simulink model "dsp_blr_hikaku_nakamura_futagi"  (R2018a)
settings: Solver=VariableStepAuto  StartTime=0.0  StopTime=100e-6  RelTol=1e-3
values from neighbouring files (symbols this model uses):
  BASELINE = 0    [dsp_blr.mat]
libraries: xbsIndex_r4 x934, xrbsSSR_Library x35, simulink x3, dspsigattribs x2, hdlsllib x2
(part 2 of 6)

== system dsp_blr_hikaku_nakamura_futagi/+cut ==
  In1 : Inport
  AddSub7 : xbsIndex_r4/AddSub  mode=Subtraction  use_carryin=off  use_carryout=off  en=off  latency=0  precision=User Defined  arith_type="Signed  (2's comp)"  n_bits=17  bin_pt=4  quantization=Truncate  overflow=Wrap  use_behavioral_HDL=off  hw_selection=Fabric  pipelined=off  dbl_ovrd=off  block_type=addsub
  Delay2 : xbsIndex_r4/Delay  rst=off  infoeditControl=Selection of Reset will increase slice count due to use of real FFs and instead of SRLs  en=off  latency=1  reg_retiming=off  dbl_ovrd=off  block_type=delay
  Delay3 : xbsIndex_r4/Delay  rst=off  infoeditControl=Selection of Reset will increase slice count due to use of real FFs and instead of SRLs  en=off  latency=3  reg_retiming=off  dbl_ovrd=off  block_type=delay
  P*e[n] : xbsIndex_r4/Mult  precision=Full  arith_type="Signed  (2's comp)"  n_bits=16  bin_pt=14  quantization=Truncate  overflow=Wrap  en=off  latency=3  use_behavioral_HDL=off  opt=Speed  use_embedded=on  optimum_pipeline=off  pipeline=on  dbl_ovrd=off  use_rpm=on  placement_style=Triangular  block_type=mult
  Shift7 : xbsIndex_r4/Shift  shift_dir=Right  shift_bits=1  en=off  latency=1  precision=Full  arith_type="Signed  (2's comp)"  n_bits=16  bin_pt=14  quantization=Truncate  overflow=Wrap  dbl_ovrd=off  block_type=shift
  Threshold : xbsIndex_r4/Threshold  en=off  latency=1  dbl_ovrd=off  block_type=sgn
      settings: infoedit="Presents -1 as output if input is negative; otherwise presents 1.  Output is a two bit signed number."
  Out1 : Outport
  wires:
  Shift7/1 -> Out1/1
  Delay2/1 -> P*e[n]/1, Delay3/1
  In1/1 -> Threshold/1, Delay2/1
  Threshold/1 -> P*e[n]/2
  Delay3/1 -> AddSub7/1
  AddSub7/1 -> Shift7/1
  P*e[n]/1 -> AddSub7/2

== system dsp_blr_hikaku_nakamura_futagi/8sample_average 1 ==
  valid_in : Inport
  data_in : Inport  Port=2
  Vector_sum : Subsystem
  scaling : Subsystem
  ave_valid_out : Outport
  ave_data_out : Outport  Port=2
  wires:
  valid_in/1 -> scaling/1(valid_in)
  Vector_sum/1(sum_data_out) -> scaling/2(data_in)
  scaling/2(data_out) -> ave_data_out/1
  data_in/1 -> Vector_sum/1(tdata_in)
  scaling/1(valid_out) -> ave_valid_out/1

== system dsp_blr_hikaku_nakamura_futagi/8sample_average 3 ==
  valid_in : Inport
  data_in : Inport  Port=2
  Vector_sum : Subsystem
  scaling : Subsystem
  ave_valid_out : Outport
  ave_data_out : Outport  Port=2
  wires:
  valid_in/1 -> scaling/1(valid_in)
  Vector_sum/1(sum_data_out) -> scaling/2(data_in)
  scaling/2(data_out) -> ave_data_out/1
  data_in/1 -> Vector_sum/1(tdata_in)
  scaling/1(valid_out) -> ave_valid_out/1

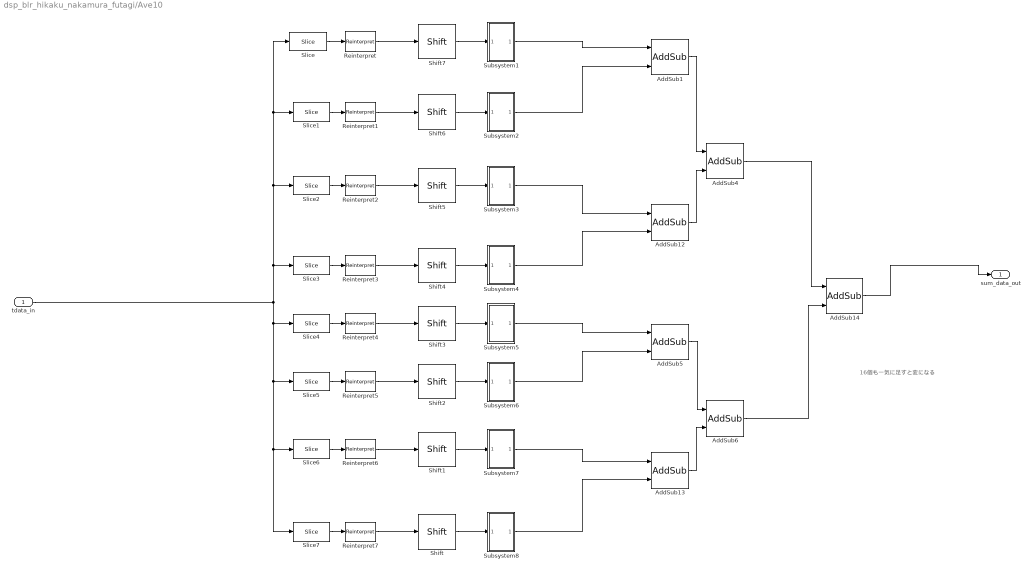
== system dsp_blr_hikaku_nakamura_futagi/Ave10 ==
  note: 16個も一気に足すと変になる
  tdata_in : Inport
  AddSub{1,12..14} (4 alike) : xbsIndex_r4/AddSub  mode=Addition  use_carryin=off  use_carryout=off  en=off  latency=0  precision=User Defined  arith_type="Signed  (2's comp)"  n_bits=17  bin_pt=4  quantization=Truncate  overflow=Wrap  use_behavioral_HDL=off  hw_selection=Fabric  pipelined=off  dbl_ovrd=off  block_type=addsub
  AddSub4 : xbsIndex_r4/AddSub  mode=Addition  use_carryin=off  use_carryout=off  en=off  latency=0  precision=Full  arith_type="Signed  (2's comp)"  n_bits=18  bin_pt=4  quantization=Truncate  overflow=Wrap  use_behavioral_HDL=off  hw_selection=Fabric  pipelined=off  dbl_ovrd=off  block_type=addsub
  AddSub5 : xbsIndex_r4/AddSub  mode=Addition  use_carryin=off  use_carryout=off  en=off  latency=0  precision=Full  arith_type="Signed  (2's comp)"  n_bits=18  bin_pt=4  quantization=Truncate  overflow=Wrap  use_behavioral_HDL=off  hw_selection=Fabric  pipelined=off  dbl_ovrd=off  block_type=addsub
  AddSub6 : xbsIndex_r4/AddSub  mode=Addition  use_carryin=off  use_carryout=off  en=off  latency=0  precision=User Defined  arith_type="Signed  (2's comp)"  n_bits=19  bin_pt=4  quantization=Truncate  overflow=Wrap  use_behavioral_HDL=off  hw_selection=Fabric  pipelined=off  dbl_ovrd=off  block_type=addsub
  Reinterpret{,1..7} (8 alike) : xbsIndex_r4/Reinterpret  force_arith_type=on  arith_type="Signed  (2's comp)"  force_bin_pt=on  bin_pt=4  block_type=reinterpret
  Shift{,1..7} (8 alike) : xbsIndex_r4/Shift  shift_dir=Right  shift_bits=6  en=off  latency=1  precision=Full  arith_type="Signed  (2's comp)"  n_bits=16  bin_pt=14  quantization=Truncate  overflow=Wrap  dbl_ovrd=off  block_type=shift
  Slice : xbsIndex_r4/Slice  nbits=16  boolean_output=off  mode=Two Bit Locations  bit1=15  base1=LSB of Input  bit0=0  base0=LSB of Input  dbl_ovrd=off  block_type=slice
  Slice1 : xbsIndex_r4/Slice  nbits=16  boolean_output=off  mode=Two Bit Locations  bit1=31  base1=LSB of Input  bit0=16  base0=LSB of Input  dbl_ovrd=off  block_type=slice
  Slice2 : xbsIndex_r4/Slice  nbits=16  boolean_output=off  mode=Two Bit Locations  bit1=47  base1=LSB of Input  bit0=32  base0=LSB of Input  dbl_ovrd=off  block_type=slice
  Slice3 : xbsIndex_r4/Slice  nbits=16  boolean_output=off  mode=Two Bit Locations  bit1=63  base1=LSB of Input  bit0=48  base0=LSB of Input  dbl_ovrd=off  block_type=slice
  Slice4 : xbsIndex_r4/Slice  nbits=16  boolean_output=off  mode=Two Bit Locations  bit1=79  base1=LSB of Input  bit0=64  base0=LSB of Input  dbl_ovrd=off  block_type=slice
  Slice5 : xbsIndex_r4/Slice  nbits=16  boolean_output=off  mode=Two Bit Locations  bit1=95  base1=LSB of Input  bit0=80  base0=LSB of Input  dbl_ovrd=off  block_type=slice
  Slice6 : xbsIndex_r4/Slice  nbits=16  boolean_output=off  mode=Two Bit Locations  bit1=111  base1=LSB of Input  bit0=96  base0=LSB of Input  dbl_ovrd=off  block_type=slice
  Slice7 : xbsIndex_r4/Slice  nbits=16  boolean_output=off  mode=Two Bit Locations  bit1=127  base1=LSB of Input  bit0=112  base0=LSB of Input  dbl_ovrd=off  block_type=slice
  Subsystem1 : Subsystem
  Subsystem2 : Subsystem
  Subsystem3 : Subsystem
  Subsystem4 : Subsystem
  Subsystem5 : Subsystem
  Subsystem6 : Subsystem
  Subsystem7 : Subsystem
  Subsystem8 : Subsystem
  sum_data_out : Outport  OutDataTypeStr=fixdt(1,19,4)
  wires:
  AddSub14/1 -> sum_data_out/1
  Reinterpret5/1 -> Shift2/1
  Reinterpret4/1 -> Shift3/1
  Reinterpret7/1 -> Shift/1
  Reinterpret3/1 -> Shift4/1
  Reinterpret2/1 -> Shift5/1
  Reinterpret1/1 -> Shift6/1
  Reinterpret/1 -> Shift7/1
  Slice7/1 -> Reinterpret7/1
  Slice6/1 -> Reinterpret6/1
  Slice5/1 -> Reinterpret5/1
  Slice4/1 -> Reinterpret4/1
  Slice3/1 -> Reinterpret3/1
  Slice2/1 -> Reinterpret2/1
  Slice1/1 -> Reinterpret1/1
  Slice/1 -> Reinterpret/1
  Subsystem5/1(Out1) -> AddSub5/1
  Subsystem6/1(Out1) -> AddSub5/2
  tdata_in/1 -> Slice3/1, Slice1/1, Slice/1, Slice2/1, Slice4/1, Slice5/1, Slice6/1, Slice7/1
  Reinterpret6/1 -> Shift1/1
  Subsystem3/1(Out1) -> AddSub12/1
  Subsystem4/1(Out1) -> AddSub12/2
  Subsystem7/1(Out1) -> AddSub13/1
  Subsystem8/1(Out1) -> AddSub13/2
  AddSub13/1 -> AddSub6/2
  AddSub5/1 -> AddSub6/1
  AddSub1/1 -> AddSub4/1
  AddSub12/1 -> AddSub4/2
  AddSub4/1 -> AddSub14/1
  AddSub6/1 -> AddSub14/2
  Shift/1 -> Subsystem8/1(In1)
  Shift1/1 -> Subsystem7/1(In1)
  Shift2/1 -> Subsystem6/1(In1)
  Shift3/1 -> Subsystem5/1(In1)
  Shift4/1 -> Subsystem4/1(In1)
  Shift5/1 -> Subsystem3/1(In1)
  Shift6/1 -> Subsystem2/1(In1)
  Shift7/1 -> Subsystem1/1(In1)
  Subsystem1/1(Out1) -> AddSub1/1
  Subsystem2/1(Out1) -> AddSub1/2

== system dsp_blr_hikaku_nakamura_futagi/Ave11 ==
  note: 16個も一気に足すと変になる
  tdata_in : Inport
  AddSub14 : xbsIndex_r4/AddSub  mode=Addition  use_carryin=off  use_carryout=off  en=off  latency=0  precision=User Defined  arith_type="Signed  (2's comp)"  n_bits=17  bin_pt=4  quantization=Truncate  overflow=Wrap  use_behavioral_HDL=off  hw_selection=Fabric  pipelined=off  dbl_ovrd=off  block_type=addsub
  AddSub4 : xbsIndex_r4/AddSub  mode=Addition  use_carryin=off  use_carryout=off  en=off  latency=0  precision=Full  arith_type="Signed  (2's comp)"  n_bits=18  bin_pt=4  quantization=Truncate  overflow=Wrap  use_behavioral_HDL=off  hw_selection=Fabric  pipelined=off  dbl_ovrd=off  block_type=addsub
  AddSub6 : xbsIndex_r4/AddSub  mode=Addition  use_carryin=off  use_carryout=off  en=off  latency=0  precision=User Defined  arith_type="Signed  (2's comp)"  n_bits=19  bin_pt=4  quantization=Truncate  overflow=Wrap  use_behavioral_HDL=off  hw_selection=Fabric  pipelined=off  dbl_ovrd=off  block_type=addsub
  Reinterpret{,2,4,6} (4 alike) : xbsIndex_r4/Reinterpret  force_arith_type=on  arith_type="Signed  (2's comp)"  force_bin_pt=on  bin_pt=4  block_type=reinterpret
  Shift{2,4,6..7} (4 alike) : xbsIndex_r4/Shift  shift_dir=Right  shift_bits=6  en=off  latency=1  precision=Full  arith_type="Signed  (2's comp)"  n_bits=16  bin_pt=14  quantization=Truncate  overflow=Wrap  dbl_ovrd=off  block_type=shift
  Slice : xbsIndex_r4/Slice  nbits=16  boolean_output=off  mode=Two Bit Locations  bit1=15  base1=LSB of Input  bit0=0  base0=LSB of Input  dbl_ovrd=off  block_type=slice
  Slice2 : xbsIndex_r4/Slice  nbits=16  boolean_output=off  mode=Two Bit Locations  bit1=47  base1=LSB of Input  bit0=32  base0=LSB of Input  dbl_ovrd=off  block_type=slice
  Slice4 : xbsIndex_r4/Slice  nbits=16  boolean_output=off  mode=Two Bit Locations  bit1=79  base1=LSB of Input  bit0=64  base0=LSB of Input  dbl_ovrd=off  block_type=slice
  Slice6 : xbsIndex_r4/Slice  nbits=16  boolean_output=off  mode=Two Bit Locations  bit1=111  base1=LSB of Input  bit0=96  base0=LSB of Input  dbl_ovrd=off  block_type=slice
  Subsystem1 : Subsystem
  Subsystem3 : Subsystem
  Subsystem5 : Subsystem
  Subsystem7 : Subsystem
  sum_data_out : Outport  OutDataTypeStr=fixdt(1,19,4)
  wires:
  AddSub14/1 -> sum_data_out/1
  Reinterpret4/1 -> Shift4/1
  Reinterpret2/1 -> Shift2/1
  Reinterpret/1 -> Shift7/1
  Slice6/1 -> Reinterpret6/1
  Slice4/1 -> Reinterpret4/1
  Slice2/1 -> Reinterpret2/1
  Slice/1 -> Reinterpret/1
  tdata_in/1 -> Slice/1, Slice2/1, Slice4/1, Slice6/1
  Reinterpret6/1 -> Shift6/1
  Subsystem7/1(Out1) -> AddSub6/2
  Subsystem5/1(Out1) -> AddSub6/1
  Subsystem1/1(Out1) -> AddSub4/1
  Subsystem3/1(Out1) -> AddSub4/2
  AddSub4/1 -> AddSub14/1
  AddSub6/1 -> AddSub14/2
  Shift6/1 -> Subsystem7/1(In1)
  Shift4/1 -> Subsystem5/1(In1)
  Shift2/1 -> Subsystem3/1(In1)
  Shift7/1 -> Subsystem1/1(In1)

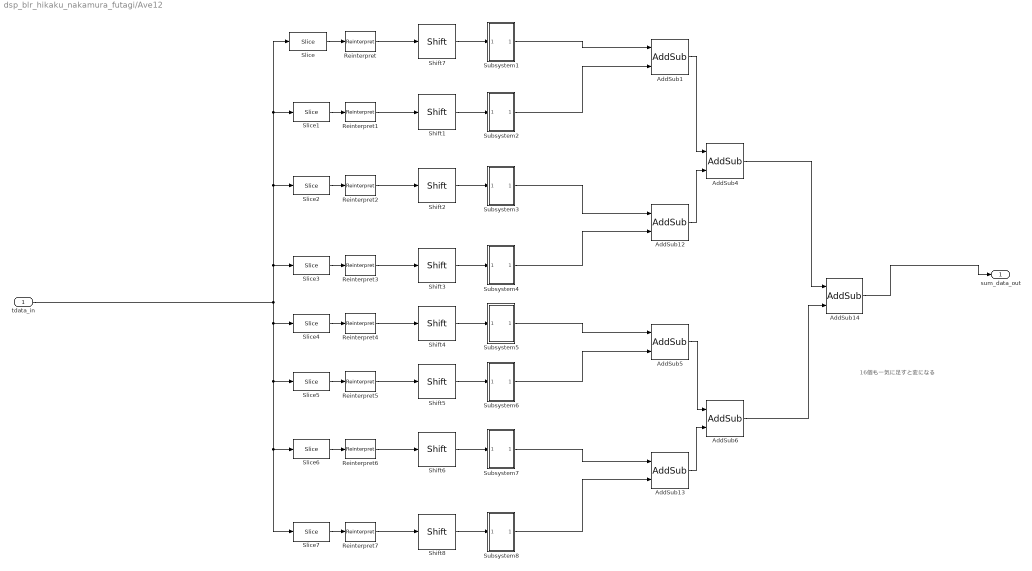
== system dsp_blr_hikaku_nakamura_futagi/Ave12 ==
  note: 16個も一気に足すと変になる
  tdata_in : Inport
  AddSub{1,12..14} (4 alike) : xbsIndex_r4/AddSub  mode=Addition  use_carryin=off  use_carryout=off  en=off  latency=0  precision=User Defined  arith_type="Signed  (2's comp)"  n_bits=17  bin_pt=4  quantization=Truncate  overflow=Wrap  use_behavioral_HDL=off  hw_selection=Fabric  pipelined=off  dbl_ovrd=off  block_type=addsub
  AddSub4 : xbsIndex_r4/AddSub  mode=Addition  use_carryin=off  use_carryout=off  en=off  latency=0  precision=Full  arith_type="Signed  (2's comp)"  n_bits=18  bin_pt=4  quantization=Truncate  overflow=Wrap  use_behavioral_HDL=off  hw_selection=Fabric  pipelined=off  dbl_ovrd=off  block_type=addsub
  AddSub5 : xbsIndex_r4/AddSub  mode=Addition  use_carryin=off  use_carryout=off  en=off  latency=0  precision=Full  arith_type="Signed  (2's comp)"  n_bits=18  bin_pt=4  quantization=Truncate  overflow=Wrap  use_behavioral_HDL=off  hw_selection=Fabric  pipelined=off  dbl_ovrd=off  block_type=addsub
  AddSub6 : xbsIndex_r4/AddSub  mode=Addition  use_carryin=off  use_carryout=off  en=off  latency=0  precision=User Defined  arith_type="Signed  (2's comp)"  n_bits=19  bin_pt=4  quantization=Truncate  overflow=Wrap  use_behavioral_HDL=off  hw_selection=Fabric  pipelined=off  dbl_ovrd=off  block_type=addsub
  Reinterpret{,1..7} (8 alike) : xbsIndex_r4/Reinterpret  force_arith_type=on  arith_type="Signed  (2's comp)"  force_bin_pt=on  bin_pt=4  block_type=reinterpret
  Shift{1..8} (8 alike) : xbsIndex_r4/Shift  shift_dir=Right  shift_bits=7  en=off  latency=1  precision=Full  arith_type="Signed  (2's comp)"  n_bits=16  bin_pt=14  quantization=Truncate  overflow=Wrap  dbl_ovrd=off  block_type=shift
  Slice : xbsIndex_r4/Slice  nbits=16  boolean_output=off  mode=Two Bit Locations  bit1=15  base1=LSB of Input  bit0=0  base0=LSB of Input  dbl_ovrd=off  block_type=slice
  Slice1 : xbsIndex_r4/Slice  nbits=16  boolean_output=off  mode=Two Bit Locations  bit1=31  base1=LSB of Input  bit0=16  base0=LSB of Input  dbl_ovrd=off  block_type=slice
  Slice2 : xbsIndex_r4/Slice  nbits=16  boolean_output=off  mode=Two Bit Locations  bit1=47  base1=LSB of Input  bit0=32  base0=LSB of Input  dbl_ovrd=off  block_type=slice
  Slice3 : xbsIndex_r4/Slice  nbits=16  boolean_output=off  mode=Two Bit Locations  bit1=63  base1=LSB of Input  bit0=48  base0=LSB of Input  dbl_ovrd=off  block_type=slice
  Slice4 : xbsIndex_r4/Slice  nbits=16  boolean_output=off  mode=Two Bit Locations  bit1=79  base1=LSB of Input  bit0=64  base0=LSB of Input  dbl_ovrd=off  block_type=slice
  Slice5 : xbsIndex_r4/Slice  nbits=16  boolean_output=off  mode=Two Bit Locations  bit1=95  base1=LSB of Input  bit0=80  base0=LSB of Input  dbl_ovrd=off  block_type=slice
  Slice6 : xbsIndex_r4/Slice  nbits=16  boolean_output=off  mode=Two Bit Locations  bit1=111  base1=LSB of Input  bit0=96  base0=LSB of Input  dbl_ovrd=off  block_type=slice
  Slice7 : xbsIndex_r4/Slice  nbits=16  boolean_output=off  mode=Two Bit Locations  bit1=127  base1=LSB of Input  bit0=112  base0=LSB of Input  dbl_ovrd=off  block_type=slice
  Subsystem1 : Subsystem
  Subsystem2 : Subsystem
  Subsystem3 : Subsystem
  Subsystem4 : Subsystem
  Subsystem5 : Subsystem
  Subsystem6 : Subsystem
  Subsystem7 : Subsystem
  Subsystem8 : Subsystem
  sum_data_out : Outport  OutDataTypeStr=fixdt(1,19,4)
  wires:
  AddSub14/1 -> sum_data_out/1
  Reinterpret5/1 -> Shift5/1
  Reinterpret4/1 -> Shift4/1
  Reinterpret7/1 -> Shift8/1
  Reinterpret3/1 -> Shift3/1
  Reinterpret2/1 -> Shift2/1
  Reinterpret1/1 -> Shift1/1
  Reinterpret/1 -> Shift7/1
  Slice7/1 -> Reinterpret7/1
  Slice6/1 -> Reinterpret6/1
  Slice5/1 -> Reinterpret5/1
  Slice4/1 -> Reinterpret4/1
  Slice3/1 -> Reinterpret3/1
  Slice2/1 -> Reinterpret2/1
  Slice1/1 -> Reinterpret1/1
  Slice/1 -> Reinterpret/1
  Subsystem5/1(Out1) -> AddSub5/1
  Subsystem6/1(Out1) -> AddSub5/2
  tdata_in/1 -> Slice3/1, Slice1/1, Slice/1, Slice2/1, Slice4/1, Slice5/1, Slice6/1, Slice7/1
  Reinterpret6/1 -> Shift6/1
  Subsystem3/1(Out1) -> AddSub12/1
  Subsystem4/1(Out1) -> AddSub12/2
  Subsystem7/1(Out1) -> AddSub13/1
  Subsystem8/1(Out1) -> AddSub13/2
  AddSub13/1 -> AddSub6/2
  AddSub5/1 -> AddSub6/1
  AddSub1/1 -> AddSub4/1
  AddSub12/1 -> AddSub4/2
  AddSub4/1 -> AddSub14/1
  AddSub6/1 -> AddSub14/2
  Shift8/1 -> Subsystem8/1(In1)
  Shift6/1 -> Subsystem7/1(In1)
  Shift5/1 -> Subsystem6/1(In1)
  Shift4/1 -> Subsystem5/1(In1)
  Shift3/1 -> Subsystem4/1(In1)
  Shift2/1 -> Subsystem3/1(In1)
  Shift1/1 -> Subsystem2/1(In1)
  Shift7/1 -> Subsystem1/1(In1)
  Subsystem1/1(Out1) -> AddSub1/1
  Subsystem2/1(Out1) -> AddSub1/2

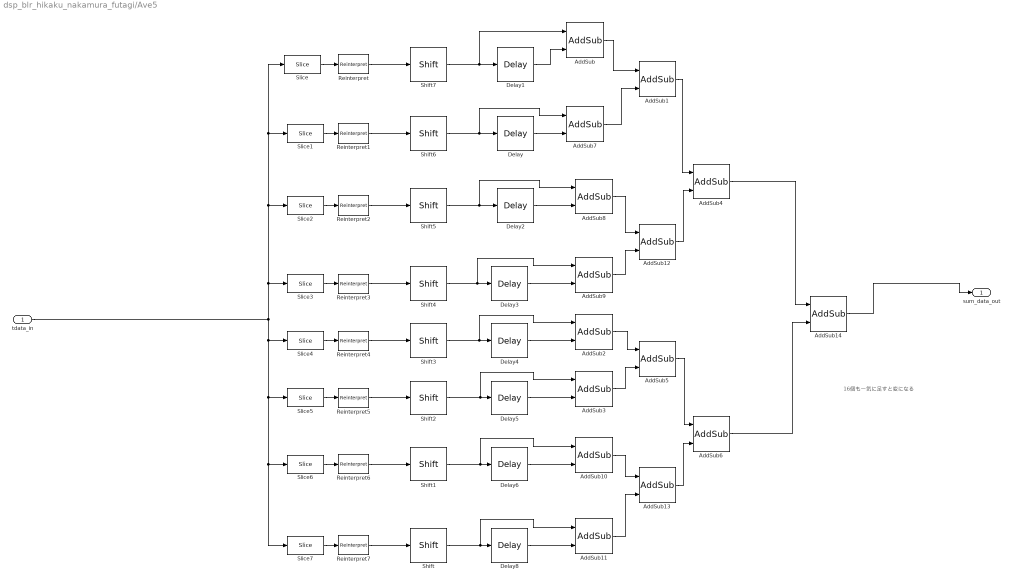
== system dsp_blr_hikaku_nakamura_futagi/Ave5 ==
  note: 16個も一気に足すと変になる
  tdata_in : Inport
  AddSub{,1..3,7..14} (12 alike) : xbsIndex_r4/AddSub  mode=Addition  use_carryin=off  use_carryout=off  en=off  latency=0  precision=User Defined  arith_type="Signed  (2's comp)"  n_bits=17  bin_pt=4  quantization=Truncate  overflow=Wrap  use_behavioral_HDL=off  hw_selection=Fabric  pipelined=off  dbl_ovrd=off  block_type=addsub
  AddSub4 : xbsIndex_r4/AddSub  mode=Addition  use_carryin=off  use_carryout=off  en=off  latency=0  precision=Full  arith_type="Signed  (2's comp)"  n_bits=18  bin_pt=4  quantization=Truncate  overflow=Wrap  use_behavioral_HDL=off  hw_selection=Fabric  pipelined=off  dbl_ovrd=off  block_type=addsub
  AddSub5 : xbsIndex_r4/AddSub  mode=Addition  use_carryin=off  use_carryout=off  en=off  latency=0  precision=Full  arith_type="Signed  (2's comp)"  n_bits=18  bin_pt=4  quantization=Truncate  overflow=Wrap  use_behavioral_HDL=off  hw_selection=Fabric  pipelined=off  dbl_ovrd=off  block_type=addsub
  AddSub6 : xbsIndex_r4/AddSub  mode=Addition  use_carryin=off  use_carryout=off  en=off  latency=0  precision=User Defined  arith_type="Signed  (2's comp)"  n_bits=19  bin_pt=4  quantization=Truncate  overflow=Wrap  use_behavioral_HDL=off  hw_selection=Fabric  pipelined=off  dbl_ovrd=off  block_type=addsub
  Delay{,1..6,8} (8 alike) : xbsIndex_r4/Delay  rst=off  infoeditControl=Selection of Reset will increase slice count due to use of real FFs and instead of SRLs  en=off  latency=1  reg_retiming=off  dbl_ovrd=off  block_type=delay
  Reinterpret{,1..7} (8 alike) : xbsIndex_r4/Reinterpret  force_arith_type=on  arith_type="Signed  (2's comp)"  force_bin_pt=on  bin_pt=4  block_type=reinterpret
  Shift{,1..7} (8 alike) : xbsIndex_r4/Shift  shift_dir=Right  shift_bits=4  en=off  latency=1  precision=Full  arith_type="Signed  (2's comp)"  n_bits=16  bin_pt=14  quantization=Truncate  overflow=Wrap  dbl_ovrd=off  block_type=shift
  Slice : xbsIndex_r4/Slice  nbits=16  boolean_output=off  mode=Two Bit Locations  bit1=15  base1=LSB of Input  bit0=0  base0=LSB of Input  dbl_ovrd=off  block_type=slice
  Slice1 : xbsIndex_r4/Slice  nbits=16  boolean_output=off  mode=Two Bit Locations  bit1=31  base1=LSB of Input  bit0=16  base0=LSB of Input  dbl_ovrd=off  block_type=slice
  Slice2 : xbsIndex_r4/Slice  nbits=16  boolean_output=off  mode=Two Bit Locations  bit1=47  base1=LSB of Input  bit0=32  base0=LSB of Input  dbl_ovrd=off  block_type=slice
  Slice3 : xbsIndex_r4/Slice  nbits=16  boolean_output=off  mode=Two Bit Locations  bit1=63  base1=LSB of Input  bit0=48  base0=LSB of Input  dbl_ovrd=off  block_type=slice
  Slice4 : xbsIndex_r4/Slice  nbits=16  boolean_output=off  mode=Two Bit Locations  bit1=79  base1=LSB of Input  bit0=64  base0=LSB of Input  dbl_ovrd=off  block_type=slice
  Slice5 : xbsIndex_r4/Slice  nbits=16  boolean_output=off  mode=Two Bit Locations  bit1=95  base1=LSB of Input  bit0=80  base0=LSB of Input  dbl_ovrd=off  block_type=slice
  Slice6 : xbsIndex_r4/Slice  nbits=16  boolean_output=off  mode=Two Bit Locations  bit1=111  base1=LSB of Input  bit0=96  base0=LSB of Input  dbl_ovrd=off  block_type=slice
  Slice7 : xbsIndex_r4/Slice  nbits=16  boolean_output=off  mode=Two Bit Locations  bit1=127  base1=LSB of Input  bit0=112  base0=LSB of Input  dbl_ovrd=off  block_type=slice
  sum_data_out : Outport  OutDataTypeStr=fixdt(1,19,4)
  wires:
  AddSub14/1 -> sum_data_out/1
  Delay5/1 -> AddSub3/2
  Reinterpret5/1 -> Shift2/1
  Delay4/1 -> AddSub2/2
  Reinterpret4/1 -> Shift3/1
  AddSub7/1 -> AddSub1/2
  AddSub/1 -> AddSub1/1
  Reinterpret7/1 -> Shift/1
  Reinterpret3/1 -> Shift4/1
  Reinterpret2/1 -> Shift5/1
  Reinterpret1/1 -> Shift6/1
  Reinterpret/1 -> Shift7/1
  Slice7/1 -> Reinterpret7/1
  Slice6/1 -> Reinterpret6/1
  Slice5/1 -> Reinterpret5/1
  Slice4/1 -> Reinterpret4/1
  Slice3/1 -> Reinterpret3/1
  Slice2/1 -> Reinterpret2/1
  Slice1/1 -> Reinterpret1/1
  Slice/1 -> Reinterpret/1
  AddSub2/1 -> AddSub5/1
  AddSub3/1 -> AddSub5/2
  tdata_in/1 -> Slice3/1, Slice1/1, Slice/1, Slice2/1, Slice4/1, Slice5/1, Slice6/1, Slice7/1
  Delay1/1 -> AddSub/2
  Delay/1 -> AddSub7/2
  Delay2/1 -> AddSub8/2
  Delay3/1 -> AddSub9/2
  Delay6/1 -> AddSub10/2
  Reinterpret6/1 -> Shift1/1
  Delay8/1 -> AddSub11/2
  AddSub8/1 -> AddSub12/1
  AddSub9/1 -> AddSub12/2
  AddSub10/1 -> AddSub13/1
  AddSub11/1 -> AddSub13/2
  AddSub13/1 -> AddSub6/2
  AddSub5/1 -> AddSub6/1
  AddSub1/1 -> AddSub4/1
  AddSub12/1 -> AddSub4/2
  AddSub4/1 -> AddSub14/1
  AddSub6/1 -> AddSub14/2
  Shift/1 -> AddSub11/1, Delay8/1
  Shift1/1 -> AddSub10/1, Delay6/1
  Shift2/1 -> AddSub3/1, Delay5/1
  Shift3/1 -> AddSub2/1, Delay4/1
  Shift4/1 -> AddSub9/1, Delay3/1
  Shift5/1 -> AddSub8/1, Delay2/1
  Shift6/1 -> AddSub7/1, Delay/1
  Shift7/1 -> AddSub/1, Delay1/1

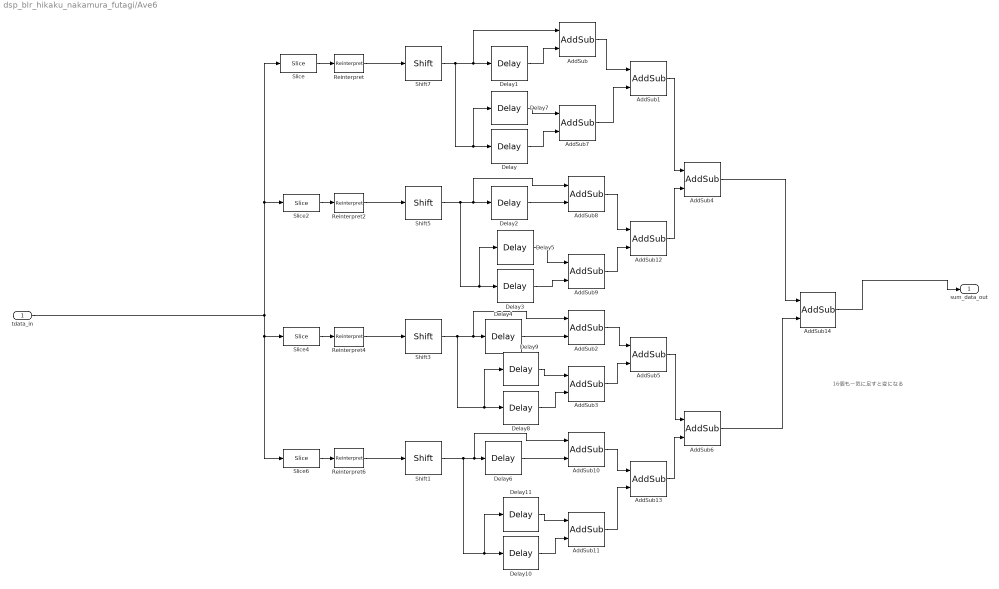
== system dsp_blr_hikaku_nakamura_futagi/Ave6 ==
  note: 16個も一気に足すと変になる
  tdata_in : Inport
  AddSub{,1..3,7..14} (12 alike) : xbsIndex_r4/AddSub  mode=Addition  use_carryin=off  use_carryout=off  en=off  latency=0  precision=User Defined  arith_type="Signed  (2's comp)"  n_bits=17  bin_pt=4  quantization=Truncate  overflow=Wrap  use_behavioral_HDL=off  hw_selection=Fabric  pipelined=off  dbl_ovrd=off  block_type=addsub
  AddSub4 : xbsIndex_r4/AddSub  mode=Addition  use_carryin=off  use_carryout=off  en=off  latency=0  precision=Full  arith_type="Signed  (2's comp)"  n_bits=18  bin_pt=4  quantization=Truncate  overflow=Wrap  use_behavioral_HDL=off  hw_selection=Fabric  pipelined=off  dbl_ovrd=off  block_type=addsub
  AddSub5 : xbsIndex_r4/AddSub  mode=Addition  use_carryin=off  use_carryout=off  en=off  latency=0  precision=Full  arith_type="Signed  (2's comp)"  n_bits=18  bin_pt=4  quantization=Truncate  overflow=Wrap  use_behavioral_HDL=off  hw_selection=Fabric  pipelined=off  dbl_ovrd=off  block_type=addsub
  AddSub6 : xbsIndex_r4/AddSub  mode=Addition  use_carryin=off  use_carryout=off  en=off  latency=0  precision=User Defined  arith_type="Signed  (2's comp)"  n_bits=19  bin_pt=4  quantization=Truncate  overflow=Wrap  use_behavioral_HDL=off  hw_selection=Fabric  pipelined=off  dbl_ovrd=off  block_type=addsub
  Delay{,3,8,10} (4 alike) : xbsIndex_r4/Delay  rst=off  infoeditControl=Selection of Reset will increase slice count due to use of real FFs and instead of SRLs  en=off  latency=3  reg_retiming=off  dbl_ovrd=off  block_type=delay
  Delay{1..2,4,6} (4 alike) : xbsIndex_r4/Delay  rst=off  infoeditControl=Selection of Reset will increase slice count due to use of real FFs and instead of SRLs  en=off  latency=1  reg_retiming=off  dbl_ovrd=off  block_type=delay
  Delay{5,7,9,11} (4 alike) : xbsIndex_r4/Delay  rst=off  infoeditControl=Selection of Reset will increase slice count due to use of real FFs and instead of SRLs  en=off  latency=2  reg_retiming=off  dbl_ovrd=off  block_type=delay
  Reinterpret{,2,4,6} (4 alike) : xbsIndex_r4/Reinterpret  force_arith_type=on  arith_type="Signed  (2's comp)"  force_bin_pt=on  bin_pt=4  block_type=reinterpret
  Shift{1,3,5,7} (4 alike) : xbsIndex_r4/Shift  shift_dir=Right  shift_bits=4  en=off  latency=1  precision=Full  arith_type="Signed  (2's comp)"  n_bits=16  bin_pt=14  quantization=Truncate  overflow=Wrap  dbl_ovrd=off  block_type=shift
  Slice : xbsIndex_r4/Slice  nbits=16  boolean_output=off  mode=Two Bit Locations  bit1=15  base1=LSB of Input  bit0=0  base0=LSB of Input  dbl_ovrd=off  block_type=slice
  Slice2 : xbsIndex_r4/Slice  nbits=16  boolean_output=off  mode=Two Bit Locations  bit1=47  base1=LSB of Input  bit0=32  base0=LSB of Input  dbl_ovrd=off  block_type=slice
  Slice4 : xbsIndex_r4/Slice  nbits=16  boolean_output=off  mode=Two Bit Locations  bit1=79  base1=LSB of Input  bit0=64  base0=LSB of Input  dbl_ovrd=off  block_type=slice
  Slice6 : xbsIndex_r4/Slice  nbits=16  boolean_output=off  mode=Two Bit Locations  bit1=111  base1=LSB of Input  bit0=96  base0=LSB of Input  dbl_ovrd=off  block_type=slice
  sum_data_out : Outport  OutDataTypeStr=fixdt(1,19,4)
  wires:
  AddSub12/1 -> AddSub4/2
  Shift7/1 -> Delay7/1, Delay/1, AddSub/1, Delay1/1
  Delay6/1 -> AddSub10/2
  Slice4/1 -> Reinterpret4/1
  AddSub8/1 -> AddSub12/1
  AddSub11/1 -> AddSub13/2
  Reinterpret6/1 -> Shift1/1
  Delay/1 -> AddSub7/2
  AddSub5/1 -> AddSub6/1
  tdata_in/1 -> Slice/1, Slice2/1, Slice4/1, Slice6/1
  AddSub4/1 -> AddSub14/1
  AddSub2/1 -> AddSub5/1
  Delay2/1 -> AddSub8/2
  AddSub9/1 -> AddSub12/2
  Slice/1 -> Reinterpret/1
  Delay1/1 -> AddSub/2
  AddSub13/1 -> AddSub6/2
  AddSub14/1 -> sum_data_out/1
  AddSub10/1 -> AddSub13/1
  Slice2/1 -> Reinterpret2/1
  Slice6/1 -> Reinterpret6/1
  Reinterpret4/1 -> Shift3/1
  AddSub7/1 -> AddSub1/2
  Delay4/1 -> AddSub2/2
  AddSub6/1 -> AddSub14/2
  AddSub/1 -> AddSub1/1
  AddSub3/1 -> AddSub5/2
  AddSub1/1 -> AddSub4/1
  Reinterpret2/1 -> Shift5/1
  Reinterpret/1 -> Shift7/1
  Delay7/1 -> AddSub7/1
  Delay3/1 -> AddSub9/2
  Shift5/1 -> Delay5/1, Delay3/1, AddSub8/1, Delay2/1
  Delay5/1 -> AddSub9/1
  Delay8/1 -> AddSub3/2
  Shift3/1 -> Delay9/1, Delay8/1, AddSub2/1, Delay4/1
  Delay9/1 -> AddSub3/1
  Delay10/1 -> AddSub11/2
  Shift1/1 -> Delay11/1, Delay10/1, AddSub10/1, Delay6/1
  Delay11/1 -> AddSub11/1

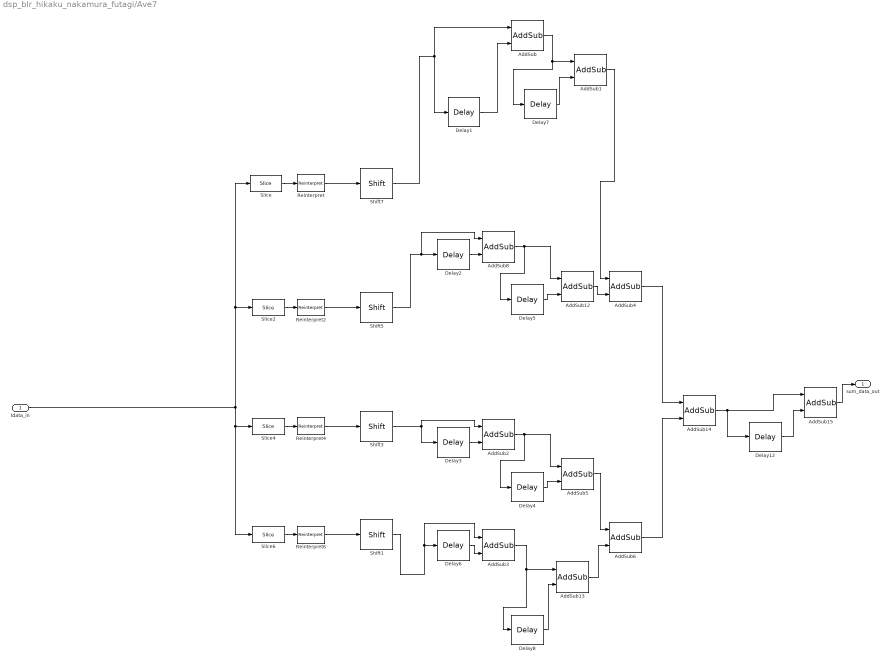
== system dsp_blr_hikaku_nakamura_futagi/Ave7 ==
  tdata_in : Inport
  AddSub{,1..3,8,12..15} (9 alike) : xbsIndex_r4/AddSub  mode=Addition  use_carryin=off  use_carryout=off  en=off  latency=0  precision=User Defined  arith_type="Signed  (2's comp)"  n_bits=17  bin_pt=4  quantization=Truncate  overflow=Wrap  use_behavioral_HDL=off  hw_selection=Fabric  pipelined=off  dbl_ovrd=off  block_type=addsub
  AddSub4 : xbsIndex_r4/AddSub  mode=Addition  use_carryin=off  use_carryout=off  en=off  latency=0  precision=Full  arith_type="Signed  (2's comp)"  n_bits=18  bin_pt=4  quantization=Truncate  overflow=Wrap  use_behavioral_HDL=off  hw_selection=Fabric  pipelined=off  dbl_ovrd=off  block_type=addsub
  AddSub5 : xbsIndex_r4/AddSub  mode=Addition  use_carryin=off  use_carryout=off  en=off  latency=0  precision=Full  arith_type="Signed  (2's comp)"  n_bits=18  bin_pt=4  quantization=Truncate  overflow=Wrap  use_behavioral_HDL=off  hw_selection=Fabric  pipelined=off  dbl_ovrd=off  block_type=addsub
  AddSub6 : xbsIndex_r4/AddSub  mode=Addition  use_carryin=off  use_carryout=off  en=off  latency=0  precision=User Defined  arith_type="Signed  (2's comp)"  n_bits=19  bin_pt=4  quantization=Truncate  overflow=Wrap  use_behavioral_HDL=off  hw_selection=Fabric  pipelined=off  dbl_ovrd=off  block_type=addsub
  Delay{1..3,6} (4 alike) : xbsIndex_r4/Delay  rst=off  infoeditControl=Selection of Reset will increase slice count due to use of real FFs and instead of SRLs  en=off  latency=1  reg_retiming=off  dbl_ovrd=off  block_type=delay
  Delay12 : xbsIndex_r4/Delay  rst=off  infoeditControl=Selection of Reset will increase slice count due to use of real FFs and instead of SRLs  en=off  latency=4  reg_retiming=off  dbl_ovrd=off  block_type=delay
  Delay{4..5,7..8} (4 alike) : xbsIndex_r4/Delay  rst=off  infoeditControl=Selection of Reset will increase slice count due to use of real FFs and instead of SRLs  en=off  latency=2  reg_retiming=off  dbl_ovrd=off  block_type=delay
  Reinterpret{,2,4,6} (4 alike) : xbsIndex_r4/Reinterpret  force_arith_type=on  arith_type="Signed  (2's comp)"  force_bin_pt=on  bin_pt=4  block_type=reinterpret
  Shift{1,3,5,7} (4 alike) : xbsIndex_r4/Shift  shift_dir=Right  shift_bits=5  en=off  latency=1  precision=Full  arith_type="Signed  (2's comp)"  n_bits=16  bin_pt=14  quantization=Truncate  overflow=Wrap  dbl_ovrd=off  block_type=shift
  Slice : xbsIndex_r4/Slice  nbits=16  boolean_output=off  mode=Two Bit Locations  bit1=15  base1=LSB of Input  bit0=0  base0=LSB of Input  dbl_ovrd=off  block_type=slice
  Slice2 : xbsIndex_r4/Slice  nbits=16  boolean_output=off  mode=Two Bit Locations  bit1=47  base1=LSB of Input  bit0=32  base0=LSB of Input  dbl_ovrd=off  block_type=slice
  Slice4 : xbsIndex_r4/Slice  nbits=16  boolean_output=off  mode=Two Bit Locations  bit1=79  base1=LSB of Input  bit0=64  base0=LSB of Input  dbl_ovrd=off  block_type=slice
  Slice6 : xbsIndex_r4/Slice  nbits=16  boolean_output=off  mode=Two Bit Locations  bit1=111  base1=LSB of Input  bit0=96  base0=LSB of Input  dbl_ovrd=off  block_type=slice
  sum_data_out : Outport  OutDataTypeStr=fixdt(1,19,4)
  wires:
  AddSub4/1 -> AddSub14/1
  Slice4/1 -> Reinterpret4/1
  Reinterpret6/1 -> Shift1/1
  Reinterpret2/1 -> Shift5/1
  Delay7/1 -> AddSub1/2
  AddSub1/1 -> AddSub4/1
  AddSub3/1 -> Delay8/1, AddSub13/1
  Delay8/1 -> AddSub13/2
  Delay4/1 -> AddSub5/2
  AddSub15/1 -> sum_data_out/1
  Delay6/1 -> AddSub3/2
  Shift3/1 -> Delay3/1, AddSub2/1
  tdata_in/1 -> Slice/1, Slice2/1, Slice4/1, Slice6/1
  Shift5/1 -> AddSub8/1, Delay2/1
  AddSub8/1 -> Delay5/1, AddSub12/1
  Delay12/1 -> AddSub15/2
  Slice2/1 -> Reinterpret2/1
  AddSub12/1 -> AddSub4/2
  Reinterpret/1 -> Shift7/1
  Reinterpret4/1 -> Shift3/1
  AddSub13/1 -> AddSub6/2
  Slice/1 -> Reinterpret/1
  Delay1/1 -> AddSub/2
  Slice6/1 -> Reinterpret6/1
  AddSub/1 -> Delay7/1, AddSub1/1
  Delay3/1 -> AddSub2/2
  AddSub5/1 -> AddSub6/1
  AddSub2/1 -> AddSub5/1, Delay4/1
  Shift1/1 -> AddSub3/1, Delay6/1
  Delay2/1 -> AddSub8/2
  Delay5/1 -> AddSub12/2
  AddSub14/1 -> Delay12/1, AddSub15/1
  Shift7/1 -> AddSub/1, Delay1/1
  AddSub6/1 -> AddSub14/2

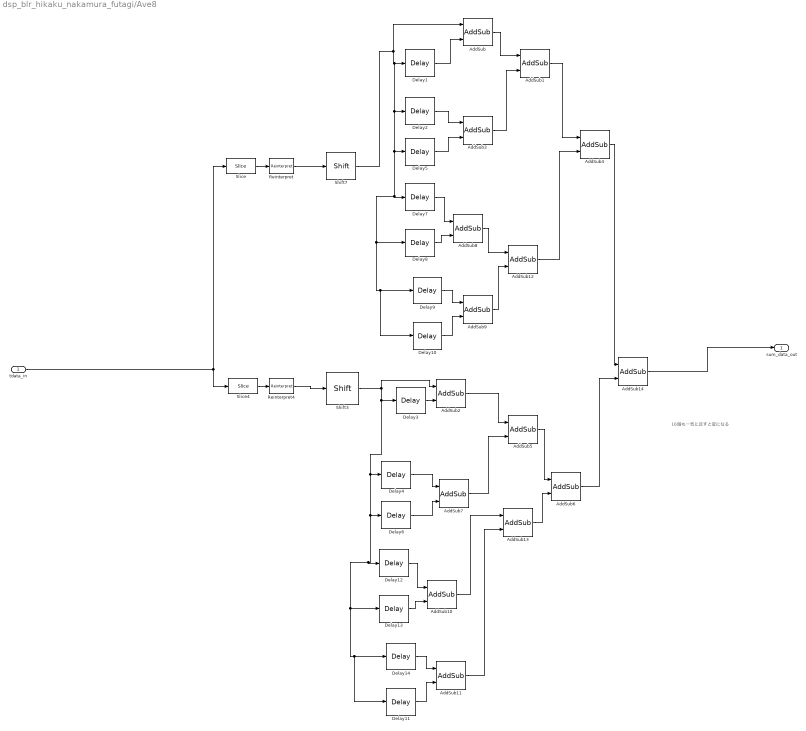
== system dsp_blr_hikaku_nakamura_futagi/Ave8 ==
  note: 16個も一気に足すと変になる
  tdata_in : Inport
  AddSub{,1..3,7..14} (12 alike) : xbsIndex_r4/AddSub  mode=Addition  use_carryin=off  use_carryout=off  en=off  latency=0  precision=User Defined  arith_type="Signed  (2's comp)"  n_bits=17  bin_pt=4  quantization=Truncate  overflow=Wrap  use_behavioral_HDL=off  hw_selection=Fabric  pipelined=off  dbl_ovrd=off  block_type=addsub
  AddSub4 : xbsIndex_r4/AddSub  mode=Addition  use_carryin=off  use_carryout=off  en=off  latency=0  precision=Full  arith_type="Signed  (2's comp)"  n_bits=18  bin_pt=4  quantization=Truncate  overflow=Wrap  use_behavioral_HDL=off  hw_selection=Fabric  pipelined=off  dbl_ovrd=off  block_type=addsub
  AddSub5 : xbsIndex_r4/AddSub  mode=Addition  use_carryin=off  use_carryout=off  en=off  latency=0  precision=Full  arith_type="Signed  (2's comp)"  n_bits=18  bin_pt=4  quantization=Truncate  overflow=Wrap  use_behavioral_HDL=off  hw_selection=Fabric  pipelined=off  dbl_ovrd=off  block_type=addsub
  AddSub6 : xbsIndex_r4/AddSub  mode=Addition  use_carryin=off  use_carryout=off  en=off  latency=0  precision=User Defined  arith_type="Signed  (2's comp)"  n_bits=19  bin_pt=4  quantization=Truncate  overflow=Wrap  use_behavioral_HDL=off  hw_selection=Fabric  pipelined=off  dbl_ovrd=off  block_type=addsub
  Delay1 : xbsIndex_r4/Delay  rst=off  infoeditControl=Selection of Reset will increase slice count due to use of real FFs and instead of SRLs  en=off  latency=1  reg_retiming=off  dbl_ovrd=off  block_type=delay
  Delay10 : xbsIndex_r4/Delay  rst=off  infoeditControl=Selection of Reset will increase slice count due to use of real FFs and instead of SRLs  en=off  latency=7  reg_retiming=off  dbl_ovrd=off  block_type=delay
  Delay11 : xbsIndex_r4/Delay  rst=off  infoeditControl=Selection of Reset will increase slice count due to use of real FFs and instead of SRLs  en=off  latency=7  reg_retiming=off  dbl_ovrd=off  block_type=delay
  Delay12 : xbsIndex_r4/Delay  rst=off  infoeditControl=Selection of Reset will increase slice count due to use of real FFs and instead of SRLs  en=off  latency=4  reg_retiming=off  dbl_ovrd=off  block_type=delay
  Delay13 : xbsIndex_r4/Delay  rst=off  infoeditControl=Selection of Reset will increase slice count due to use of real FFs and instead of SRLs  en=off  latency=5  reg_retiming=off  dbl_ovrd=off  block_type=delay
  Delay14 : xbsIndex_r4/Delay  rst=off  infoeditControl=Selection of Reset will increase slice count due to use of real FFs and instead of SRLs  en=off  latency=6  reg_retiming=off  dbl_ovrd=off  block_type=delay
  Delay2 : xbsIndex_r4/Delay  rst=off  infoeditControl=Selection of Reset will increase slice count due to use of real FFs and instead of SRLs  en=off  latency=2  reg_retiming=off  dbl_ovrd=off  block_type=delay
  Delay3 : xbsIndex_r4/Delay  rst=off  infoeditControl=Selection of Reset will increase slice count due to use of real FFs and instead of SRLs  en=off  latency=1  reg_retiming=off  dbl_ovrd=off  block_type=delay
  Delay4 : xbsIndex_r4/Delay  rst=off  infoeditControl=Selection of Reset will increase slice count due to use of real FFs and instead of SRLs  en=off  latency=2  reg_retiming=off  dbl_ovrd=off  block_type=delay
  Delay5 : xbsIndex_r4/Delay  rst=off  infoeditControl=Selection of Reset will increase slice count due to use of real FFs and instead of SRLs  en=off  latency=3  reg_retiming=off  dbl_ovrd=off  block_type=delay
  Delay6 : xbsIndex_r4/Delay  rst=off  infoeditControl=Selection of Reset will increase slice count due to use of real FFs and instead of SRLs  en=off  latency=3  reg_retiming=off  dbl_ovrd=off  block_type=delay
  Delay7 : xbsIndex_r4/Delay  rst=off  infoeditControl=Selection of Reset will increase slice count due to use of real FFs and instead of SRLs  en=off  latency=4  reg_retiming=off  dbl_ovrd=off  block_type=delay
  Delay8 : xbsIndex_r4/Delay  rst=off  infoeditControl=Selection of Reset will increase slice count due to use of real FFs and instead of SRLs  en=off  latency=5  reg_retiming=off  dbl_ovrd=off  block_type=delay
  Delay9 : xbsIndex_r4/Delay  rst=off  infoeditControl=Selection of Reset will increase slice count due to use of real FFs and instead of SRLs  en=off  latency=6  reg_retiming=off  dbl_ovrd=off  block_type=delay
  Reinterpret : xbsIndex_r4/Reinterpret  force_arith_type=on  arith_type="Signed  (2's comp)"  force_bin_pt=on  bin_pt=4  block_type=reinterpret
  Reinterpret4 : xbsIndex_r4/Reinterpret  force_arith_type=on  arith_type="Signed  (2's comp)"  force_bin_pt=on  bin_pt=4  block_type=reinterpret
  Shift3 : xbsIndex_r4/Shift  shift_dir=Right  shift_bits=4  en=off  latency=1  precision=Full  arith_type="Signed  (2's comp)"  n_bits=16  bin_pt=14  quantization=Truncate  overflow=Wrap  dbl_ovrd=off  block_type=shift
  Shift7 : xbsIndex_r4/Shift  shift_dir=Right  shift_bits=4  en=off  latency=1  precision=Full  arith_type="Signed  (2's comp)"  n_bits=16  bin_pt=14  quantization=Truncate  overflow=Wrap  dbl_ovrd=off  block_type=shift
  Slice : xbsIndex_r4/Slice  nbits=16  boolean_output=off  mode=Two Bit Locations  bit1=15  base1=LSB of Input  bit0=0  base0=LSB of Input  dbl_ovrd=off  block_type=slice
  Slice4 : xbsIndex_r4/Slice  nbits=16  boolean_output=off  mode=Two Bit Locations  bit1=79  base1=LSB of Input  bit0=64  base0=LSB of Input  dbl_ovrd=off  block_type=slice
  sum_data_out : Outport  OutDataTypeStr=fixdt(1,19,4)
  wires:
  AddSub9/1 -> AddSub12/2
  Delay4/1 -> AddSub7/1
  Delay14/1 -> AddSub11/1
  Delay13/1 -> AddSub10/2
  AddSub7/1 -> AddSub5/2
  Delay2/1 -> AddSub3/1
  AddSub10/1 -> AddSub13/1
  AddSub3/1 -> AddSub1/2
  AddSub6/1 -> AddSub14/2
  AddSub14/1 -> sum_data_out/1
  Delay10/1 -> AddSub9/2
  Slice4/1 -> Reinterpret4/1
  Delay3/1 -> AddSub2/2
  Delay6/1 -> AddSub7/2
  Delay9/1 -> AddSub9/1
  AddSub11/1 -> AddSub13/2
  AddSub12/1 -> AddSub4/2
  Reinterpret/1 -> Shift7/1
  Delay1/1 -> AddSub/2
  Shift3/1 -> AddSub2/1, Delay11/1, Delay14/1, Delay13/1, Delay12/1, Delay6/1, Delay4/1, Delay3/1
  AddSub/1 -> AddSub1/1
  Delay5/1 -> AddSub3/2
  Delay8/1 -> AddSub8/2
  Delay7/1 -> AddSub8/1
  Delay12/1 -> AddSub10/1
  tdata_in/1 -> Slice/1, Slice4/1
  AddSub4/1 -> AddSub14/1
  AddSub5/1 -> AddSub6/1
  Shift7/1 -> AddSub/1, Delay10/1, Delay9/1, Delay8/1, Delay7/1, Delay5/1, Delay2/1, Delay1/1
  Reinterpret4/1 -> Shift3/1
  AddSub13/1 -> AddSub6/2
  Delay11/1 -> AddSub11/2
  Slice/1 -> Reinterpret/1
  AddSub1/1 -> AddSub4/1
  AddSub8/1 -> AddSub12/1
  AddSub2/1 -> AddSub5/1

== system dsp_blr_hikaku_nakamura_futagi/Ave9 ==
  note: 16個も一気に足すと変になる
  tdata_in : Inport
  AddSub1 : xbsIndex_r4/AddSub  mode=Addition  use_carryin=off  use_carryout=off  en=off  latency=0  precision=User Defined  arith_type="Signed  (2's comp)"  n_bits=17  bin_pt=4  quantization=Truncate  overflow=Wrap  use_behavioral_HDL=off  hw_selection=Fabric  pipelined=off  dbl_ovrd=off  block_type=addsub
  AddSub14 : xbsIndex_r4/AddSub  mode=Addition  use_carryin=off  use_carryout=off  en=off  latency=0  precision=User Defined  arith_type="Signed  (2's comp)"  n_bits=17  bin_pt=4  quantization=Truncate  overflow=Wrap  use_behavioral_HDL=off  hw_selection=Fabric  pipelined=off  dbl_ovrd=off  block_type=addsub
  AddSub15 : xbsIndex_r4/AddSub  mode=Addition  use_carryin=off  use_carryout=off  en=off  latency=0  precision=User Defined  arith_type="Signed  (2's comp)"  n_bits=17  bin_pt=4  quantization=Truncate  overflow=Wrap  use_behavioral_HDL=off  hw_selection=Fabric  pipelined=off  dbl_ovrd=off  block_type=addsub
  Reinterpret{,2,4,6} (4 alike) : xbsIndex_r4/Reinterpret  force_arith_type=on  arith_type="Signed  (2's comp)"  force_bin_pt=on  bin_pt=4  block_type=reinterpret
  Shift{1,3,5,7} (4 alike) : xbsIndex_r4/Shift  shift_dir=Right  shift_bits=5  en=off  latency=1  precision=Full  arith_type="Signed  (2's comp)"  n_bits=16  bin_pt=14  quantization=Truncate  overflow=Wrap  dbl_ovrd=off  block_type=shift
  Slice : xbsIndex_r4/Slice  nbits=16  boolean_output=off  mode=Two Bit Locations  bit1=15  base1=LSB of Input  bit0=0  base0=LSB of Input  dbl_ovrd=off  block_type=slice
  Slice2 : xbsIndex_r4/Slice  nbits=16  boolean_output=off  mode=Two Bit Locations  bit1=47  base1=LSB of Input  bit0=32  base0=LSB of Input  dbl_ovrd=off  block_type=slice
  Slice4 : xbsIndex_r4/Slice  nbits=16  boolean_output=off  mode=Two Bit Locations  bit1=79  base1=LSB of Input  bit0=64  base0=LSB of Input  dbl_ovrd=off  block_type=slice
  Slice6 : xbsIndex_r4/Slice  nbits=16  boolean_output=off  mode=Two Bit Locations  bit1=111  base1=LSB of Input  bit0=96  base0=LSB of Input  dbl_ovrd=off  block_type=slice
  Subsystem : Subsystem
  Subsystem1 : Subsystem
  Subsystem2 : Subsystem
  Subsystem3 : Subsystem
  sum_data_out : Outport  OutDataTypeStr=fixdt(1,19,4)
  wires:
  Slice4/1 -> Reinterpret4/1
  Reinterpret/1 -> Shift7/1
  tdata_in/1 -> Slice2/1, Slice/1, Slice6/1, Slice4/1
  Reinterpret4/1 -> Shift3/1
  Slice/1 -> Reinterpret/1
  Slice2/1 -> Reinterpret2/1
  Reinterpret2/1 -> Shift5/1
  Shift7/1 -> Subsystem/1(In1)
  Subsystem/1(Out1) -> AddSub14/1
  Shift5/1 -> Subsystem1/1(In1)
  Subsystem1/1(Out1) -> AddSub14/2
  AddSub15/1 -> sum_data_out/1
  Subsystem3/1(Out1) -> AddSub1/1
  Shift1/1 -> Subsystem2/1(In1)
  Shift3/1 -> Subsystem3/1(In1)
  AddSub1/1 -> AddSub15/2
  AddSub14/1 -> AddSub15/1
  Reinterpret6/1 -> Shift1/1
  Slice6/1 -> Reinterpret6/1
  Subsystem2/1(Out1) -> AddSub1/2

== system dsp_blr_hikaku_nakamura_futagi/DBL_Scalar2Vector1 ==
  In1 : Inport
  Concat : xbsIndex_r4/Concat  num_inputs=8  dbl_ovrd=off  block_type=concat
  Reinterpret : xbsIndex_r4/Reinterpret  force_arith_type=on  arith_type=Unsigned  force_bin_pt=on  bin_pt=0  block_type=reinterpret
  Scalar2Vector : xrbsSSR_Library/Scalar2Vector  Width=16  sg_ssr=8  sg_ssr_prev=8  sg_ssr_name=vect_Scalar2Vector  block_type=scalar2vector_ssr
      settings: SourceProductName=Xilinx SSR Blockset
  Vector Reinterpret : xrbsSSR_Library/Vector Reinterpret  sg_ssr=8  sg_ssr_prev=8  force_arith_type=on  arith_type="Signed  (2's comp)"  force_bin_pt=on  bin_pt=4  block_type=reinterpret_ssr
      settings: SourceProductName=Xilinx SSR Blockset  infoedit="The Vector Reinterpret block Changes vector input signal type without altering the binary representation. You can change the signal between signed and unsigned, and relocate the binary point.<br><br>Hardware notes: In hardware this block costs nothing.<br><br>Example:  Suppose the input is 6 bits wide, signed, with 2 fractional bits, and the output is forced to unsigned with 0 fractional bits.  Then an input of -2.0 (1110.00 in binary 2's complement) becomes an output of 56 (111000 in binary)."
  Out1 : Outport
  wires:
  In1/1 -> Reinterpret/1
  Vector Reinterpret/1 -> Out1/1
  Reinterpret/1 -> Concat/1, Concat/2, Concat/3, Concat/4, Concat/8, Concat/7, Concat/6, Concat/5
  Concat/1 -> Scalar2Vector/1
  Scalar2Vector/1 -> Vector Reinterpret/1
